simulink model "Kinematic_control"  (R2022b)
settings: Solver=FixedStepAuto  StartTime=0.0  StopTime=T_final  FixedStep=Ts  RelTol=1e-3
values from neighbouring files (symbols this model uses):
  BDD_thresh = 0.5    [Run_model.m]
  d = 0.1    [Dynamicfcn.m]    (also in Run_model.m)
  I_single = sort(randperm(n_meas,n_attack)).'    [Run_model.m]
  kx = 15    [Run_model.m]
  ky = 15    [Run_model.m]
  max_iter = 2000    [Run_model.m]
  n_meas = 6    [Run_model.m]
  P_inp = 1e-8    (= 1e-08)    [Run_model.m]
  R_meas = 1e-4    (= 0.0001)    [Run_model.m]
  T_start_attack = .2*T_final    (= 60)    [Run_model.m]
  Ts = 0.01    [Dynamicfcn.m]    (also in Run_model.m)
  u0 = zeros(n_int,1)    [Run_model.m]
  y0 = zeros(n_meas,1)    [Run_model.m]
  z_hat0 = z_initial    [Run_model.m]
  z_initial = [theta0;x0;y0]    [Run_model.m]
undefined symbols (not defined in the file or in its folder): e
libraries: simulink x3, sharedTrackingLibrary x1
settings Model: Creator=Abelb  LastModifiedBy=Abelb

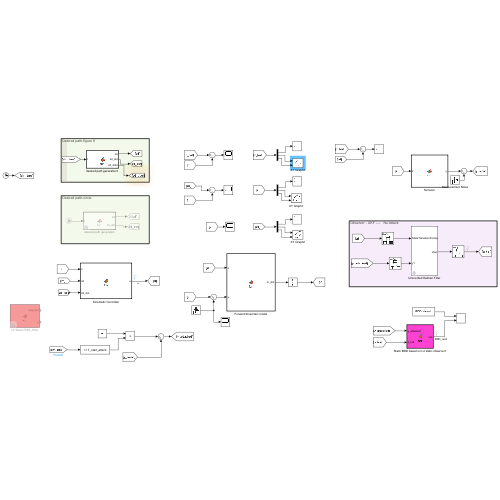
[thumbnail: Simulink's stored preview of the top-level diagram]
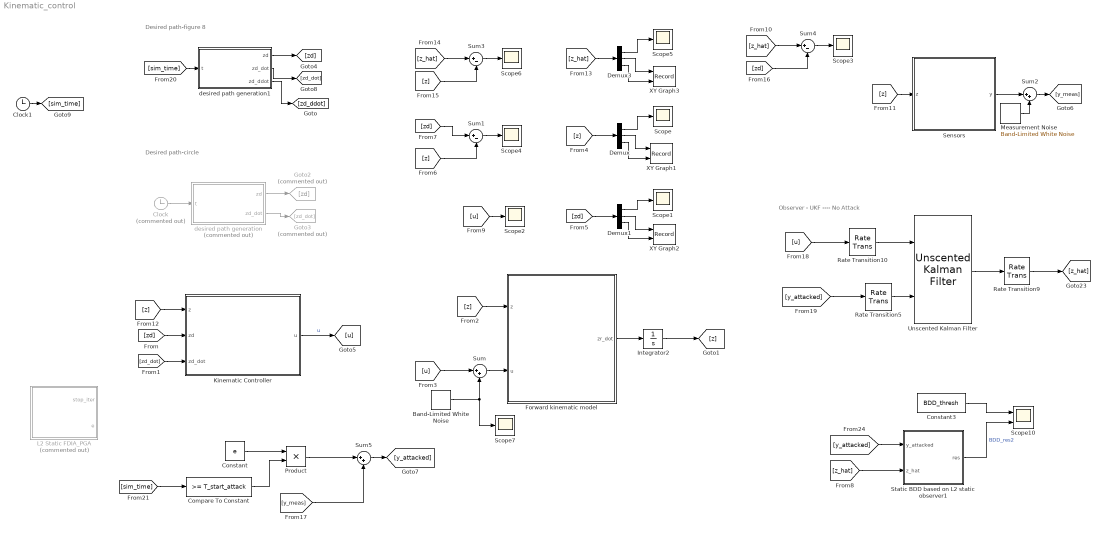
== system Kinematic_control ==
  note: Desired path-circle
  note: Desired path-figure 8
  note: Observer - UKF ---- No Attack
  Band-Limited White Noise : simulink/Sources/Band-Limited White Noise  Cov=P_inp*Ts  Ts=Ts  seed=[23341]
  Clock : Clock  Commented=on
  Clock1 : Clock
  Compare To Constant : simulink/Logic and Bit Operations/Compare To Constant  relop=>=  const=T_start_attack  OutDataTypeStr=boolean
  Constant : Constant  Value=e
  Constant3 : Constant  Value=BDD_thresh
  Demux : Demux  Outputs=3
  Demux1 : Demux  Outputs=3
  Demux3 : Demux  Outputs=3
  Forward kinematic model : MATLAB Function  TreatAsAtomicUnit=on
  Goto2 : Goto  Commented=on  GotoTag=zd
  Goto3 : Goto  Commented=on  GotoTag=zd_dot
  Integrator2 : Integrator  InitialCondition=z_initial
  Kinematic Controller : MATLAB Function  TreatAsAtomicUnit=on
  L2 Static FDIA_PGA : MATLAB Function  Commented=on  TreatAsAtomicUnit=on
  Measurement Noise : simulink/Sources/Band-Limited White Noise  Cov=R_meas*Ts  Ts=Ts  seed=[23341]
  Product : Product
  Rate Transition10 : RateTransition  InitialCondition=u0  OutPortSampleTime=Ts
  Rate Transition5 : RateTransition  InitialCondition=y0  OutPortSampleTime=Ts
  Rate Transition9 : RateTransition  InitialCondition=z_hat0  OutPortSampleTime=0
  Scope{,1..7} (8 alike) : Scope
  Scope10 : Scope  NumInputPorts=2
  Sensors : MATLAB Function  TreatAsAtomicUnit=on
  Static BDD based on L2 static observer1 : MATLAB Function  TreatAsAtomicUnit=on
  Sum : Sum  Inputs=|++
  Sum1 : Sum  Inputs=|+-
  Sum2 : Sum  Inputs=|++
  Sum3 : Sum  Inputs=|+-
  Sum4 : Sum  Inputs=|+-
  Sum5 : Sum  Inputs=|++
  Unscented Kalman Filter : sharedTrackingLibrary/Unscented Kalman Filter  StateTransitionFcn=Dynamicfcn  HasAdditiveProcessNoise=Additive  ProcessNoise=P_diag  HasTimeVaryingProcessNoise=off  HasStateTransitionFcnExtraArgument=1  InitialState=z_hat0  InitialStateCovariance=1  Alpha=1e-3  Beta=2  Kappa=0  MeasurementFcn1=measurement_model  HasMeasurementEnablePort1=off  HasAdditiveMeasurementNoise1=Additive  MeasurementNoise1=R_diag  HasTimeVaryingMeasurementNoise1=off  HasMeasurementFcnExtraArgument1=0  HasMeasurementWrapping1=off  MeasurementFcn2=myMeasurementFcn  HasMeasurementEnablePort2=off  HasAdditiveMeasurementNoise2=Additive  MeasurementNoise2=1  HasTimeVaryingMeasurementNoise2=off  HasMeasurementFcnExtraArgument2=0  HasMeasurementWrapping2=off  MeasurementFcn3=myMeasurementFcn  HasMeasurementEnablePort3=off  HasAdditiveMeasurementNoise3=Additive  MeasurementNoise3=1  HasTimeVaryingMeasurementNoise3=off  HasMeasurementFcnExtraArgument3=0  HasMeasurementWrapping3=off  MeasurementFcn4=myMeasurementFcn  HasMeasurementEnablePort4=off  HasAdditiveMeasurementNoise4=Additive  MeasurementNoise4=1  HasTimeVaryingMeasurementNoise4=off  HasMeasurementFcnExtraArgument4=0  HasMeasurementWrapping4=off  MeasurementFcn5=myMeasurementFcn  HasMeasurementEnablePort5=off  HasAdditiveMeasurementNoise5=Additive  MeasurementNoise5=1  HasTimeVaryingMeasurementNoise5=off  HasMeasurementFcnExtraArgument5=0  HasMeasurementWrapping5=off  EnableMultirate=off  StateTransitionFcnSampleTime=1  MeasurementFcn1SampleTime=1  MeasurementFcn2SampleTime=1  MeasurementFcn3SampleTime=1  MeasurementFcn4SampleTime=1  MeasurementFcn5SampleTime=1  UseCurrentEstimator=on  OutputStateCovariance=off  DataType=double  SampleTime=Ts  NumberOfMeasurements=1
      settings: LibrarySourceBlock=cstblocks/State Estimation/Unscented Kalman Filter
  XY Graph1 : Record  FileSettingsInternal="{\"entries\":[{\"content\":{\"excelSettings\":{\"content\":{},\"type\":\"Streamout.ExcelSettings\"}},\"type\":\"Streamout.FileSettingStorage\",\"uuid\":\"d8d7f9e9-d613-4e63-a397-f7a228f7e83d\"}],\"packageUris\":[\"http://schema.mathworks.com/mf0/streamout_blocks/R2020a\"],\"version\":\"1.0\"}"  Layout=[1 1]  SignalsInternal="{\"entries\":[{\"content\":{\"signals\":[{\"content\":{\"blockPath\":[\"Kinematic_control/XY Graph1\"],\"channel\":[],\"dimensions\":[1],\"domain\":\"Kinematic_control/XY Graph1\",\"lineColor\":\"#a2142f\",\"plots\":[1],\"port\":1,\"sid\":[\"\"],\"signalID\":63508,\"signalName\":\"Demux:2\"},\"type\":\"RecordBlkView.Signal\",\"uuid\":\"50b6bb6c-e09c-4804-b771-cf1436237063\"},{\"content\":{\"blockPath\":[\"Kinematic_control/XY Graph1\"],\"channel\":[],\"dimensions\":[1],\"domain\":\"Kinematic_control/XY Graph1\",\"lineColor\":\"#139fff\",\"plots\":[1],\"port\":2,\"sid\":[\"\"],\"signalID\":63512,\"signalName\":\"Demux:3\"},\"type\":\"RecordBlkView.Signal\",\"uuid\":\"32260233-ee04-4a66-bd71-a42f183323f2\"}]},\"type\":\"RecordBlkView.InputSignals\",\"uuid\":\"1d8d5054-33d6-4d2e-927d-19ce566ede83\"}],\"packageUris\":[\"http://schema.mathworks.com/mf0/streamout_blocks/R2020a\"],\"version\":\"1.0\"}"  VisualizationBindings="{\"xyplotplugin\":{\"info\":[{\"series\":[{\"bindingParametersList\":[{\"parameter\":\"X-Axis\",\"signalID\":63508,\"signalName\":\"Demux:2\"},{\"parameter\":\"Y-Axis\",\"signalID\":63512,\"signalName\":\"Demux:3\"}],\"seriesID\":26925}],\"subplotID\":1}]}}"  CompatibilityTag=XY
  XY Graph2 : Record  FileSettingsInternal="{\"entries\":[{\"content\":{\"excelSettings\":{\"content\":{},\"type\":\"Streamout.ExcelSettings\"}},\"type\":\"Streamout.FileSettingStorage\",\"uuid\":\"6c264cdc-8b0f-41a9-a26d-26fc4b96b343\"}],\"packageUris\":[\"http://schema.mathworks.com/mf0/streamout_blocks/R2020a\"],\"version\":\"1.0\"}"  Layout=[1 1]  SignalsInternal="{\"entries\":[{\"content\":{\"signals\":[{\"content\":{\"blockPath\":[\"Kinematic_control/XY Graph2\"],\"channel\":[],\"dimensions\":[1],\"domain\":\"Kinematic_control/XY Graph2\",\"lineColor\":\"#a2142f\",\"plots\":[1],\"port\":1,\"sid\":[\"\"],\"signalID\":63516,\"signalName\":\"Demux1:2\"},\"type\":\"RecordBlkView.Signal\",\"uuid\":\"dce2a075-dfc9-47ac-9e8c-4f7c2265c200\"},{\"content\":{\"blockPath\":[\"Kinematic_control/XY Graph2\"],\"channel\":[],\"dimensions\":[1],\"domain\":\"Kinematic_control/XY Graph2\",\"lineColor\":\"#139fff\",\"plots\":[1],\"port\":2,\"sid\":[\"\"],\"signalID\":63520,\"signalName\":\"Demux1:3\"},\"type\":\"RecordBlkView.Signal\",\"uuid\":\"2ac57c94-c318-4a92-bba8-431307e380f6\"}]},\"type\":\"RecordBlkView.InputSignals\",\"uuid\":\"2930b6aa-ee4b-4578-8e5b-7c11aa3c476f\"}],\"packageUris\":[\"http://schema.mathworks.com/mf0/streamout_blocks/R2020a\"],\"version\":\"1.0\"}"  VisualizationBindings="{\"xyplotplugin\":{\"info\":[{\"series\":[{\"bindingParametersList\":[{\"parameter\":\"X-Axis\",\"signalID\":63516,\"signalName\":\"Demux1:2\"},{\"parameter\":\"Y-Axis\",\"signalID\":63520,\"signalName\":\"Demux1:3\"}],\"seriesID\":33144}],\"subplotID\":1}]}}"  CompatibilityTag=XY
  XY Graph3 : Record  FileSettingsInternal="{\"entries\":[{\"content\":{\"excelSettings\":{\"content\":{},\"type\":\"Streamout.ExcelSettings\"}},\"type\":\"Streamout.FileSettingStorage\",\"uuid\":\"dbd449c8-5eee-492b-8755-63c5154b06c6\"}],\"packageUris\":[\"http://schema.mathworks.com/mf0/streamout_blocks/R2020a\"],\"version\":\"1.0\"}"  Layout=[1 1]  SignalsInternal="{\"entries\":[{\"content\":{\"signals\":[{\"content\":{\"blockPath\":[\"Kinematic_control/XY Graph3\"],\"channel\":[],\"dimensions\":[1],\"domain\":\"Kinematic_control/XY Graph3\",\"lineColor\":\"#a2142f\",\"plots\":[1],\"port\":1,\"sid\":[\"\"],\"signalID\":63524,\"signalName\":\"Demux3:2\"},\"type\":\"RecordBlkView.Signal\",\"uuid\":\"623d89f1-b4d6-49ba-b202-f47227c3b43a\"},{\"content\":{\"blockPath\":[\"Kinematic_control/XY Graph3\"],\"channel\":[],\"dimensions\":[1],\"domain\":\"Kinematic_control/XY Graph3\",\"lineColor\":\"#139fff\",\"plots\":[1],\"port\":2,\"sid\":[\"\"],\"signalID\":63528,\"signalName\":\"Demux3:3\"},\"type\":\"RecordBlkView.Signal\",\"uuid\":\"09bcd7e8-baa0-4f7a-91d9-299976939700\"}]},\"type\":\"RecordBlkView.InputSignals\",\"uuid\":\"2682f2ed-8ed1-4b26-a615-09d838c32bc9\"}],\"packageUris\":[\"http://schema.mathworks.com/mf0/streamout_blocks/R2020a\"],\"version\":\"1.0\"}"  VisualizationBindings="{\"xyplotplugin\":{\"info\":[{\"series\":[{\"bindingParametersList\":[{\"parameter\":\"X-Axis\",\"signalID\":63524,\"signalName\":\"Demux3:2\"},{\"parameter\":\"Y-Axis\",\"signalID\":63528,\"signalName\":\"Demux3:3\"}],\"seriesID\":8579}],\"subplotID\":1}]}}"  CompatibilityTag=XY
  desired path generation : MATLAB Function  Commented=on  TreatAsAtomicUnit=on
  desired path generation1 : MATLAB Function  TreatAsAtomicUnit=on
  wires:
  Forward kinematic model/1(zr_dot) -> Integrator2/1
  desired path generation1/3(zd_ddot) -> [zd_ddot]
  desired path generation1/2(zd_dot) -> [zd_dot]
  desired path generation1/1(zd) -> [zd]
  desired path generation/2(zd_dot) -> Goto3/1
  desired path generation/1(zd) -> Goto2/1
  Clock/1 -> desired path generation/1(t)
  [zd] -> Kinematic Controller/2(zd)
  [zd_dot] -> Kinematic Controller/3(zd_dot)
  Integrator2/1 -> [z]
  [z] -> Forward kinematic model/1(z)
  [z] -> Demux/1
  Demux/1 -> Scope/1
  Demux/2 -> XY Graph1/1
  Demux/3 -> XY Graph1/2
  Demux1/2 -> XY Graph2/1
  Demux1/3 -> XY Graph2/2
  [zd] -> Demux1/1
  Demux1/1 -> Scope1/1
  Kinematic Controller/1(u) -> [u]  "u"
  [zd] -> Sum1/1
  [z] -> Sum1/2
  Sum1/1 -> Scope4/1
  Unscented Kalman Filter/1 -> Rate Transition9/1
  Rate Transition9/1 -> [z_hat]
  Rate Transition10/1 -> Unscented Kalman Filter/1
  Rate Transition5/1 -> Unscented Kalman Filter/2
  [u] -> Rate Transition10/1
  [u] -> Scope2/1
  [z] -> Sensors/1(z)
  Measurement Noise/1 -> Sum2/2
  Demux3/2 -> XY Graph3/1
  Demux3/1 -> Scope5/1
  Demux3/3 -> XY Graph3/2
  [z_hat] -> Demux3/1
  [z] -> Sum3/2
  [z_hat] -> Sum3/1
  Sum3/1 -> Scope6/1
  [y_attacked] -> Rate Transition5/1
  Sensors/1(y) -> Sum2/1
  Sum2/1 -> [y_meas]
  Sum4/1 -> Scope3/1
  [zd] -> Sum4/2
  [z_hat] -> Sum4/1
  [z] -> Kinematic Controller/1(z)
  Sum/1 -> Forward kinematic model/2(u)
  [u] -> Sum/1
  Band-Limited White Noise/1 -> Scope7/1, Sum/2
  [y_meas] -> Sum5/2
  Sum5/1 -> [y_attacked]
  Product/1 -> Sum5/1
  Clock1/1 -> [sim_time]
  [sim_time] -> desired path generation1/1(t)
  [sim_time] -> Compare To Constant/1
  Compare To Constant/1 -> Product/2
  Constant/1 -> Product/1
  [y_attacked] -> Static BDD based on L2 static observer1/1(y_attacked)
  Constant3/1 -> Scope10/1
  [z_hat] -> Static BDD based on L2 static observer1/2(z_hat)
  Static BDD based on L2 static observer1/1(res) -> Scope10/2  "BDD_res2"

== matlab function Kinematic_control/desired path generation1 ==
  data: t input; zd output; zd_dot output; zd_ddot output
function [zd,zd_dot,zd_ddot] = fcn(t)

t = t/10;

a=1;
x = a*cos(t)/(1+sin(t)^2);
y = a*sin(t)*cos(t)/(1+sin(t)^2);
% unit circle (radius = 1; origin: (0,0))
zd = [atan(y./x);              % theta
      a*cos(t)/(1+sin(t)^2);         % x
      a*sin(t)*cos(t)/(1+sin(t)^2)];        % y

zd_dot = [ 0;
          -a*sin(t)*(cos(t)^2+2)/(1+sin(t)^2)^2;
          (a*cos(t)^2-2*a*sin(t)^2)/(1+sin(t)^2)^2];

z1 = (a*sin(t)^2*cos(t)^3-11*a*cos(t)^3+8*a*cos(t))/(1+sin(t)^2)^3;
z2 = -2*a*sin(t)*cos(t)*(3+2*cos(t)^2-sin(t)^2)/(1+sin(t)^2)^3;
zd_ddot = [z1;
           z2];

== matlab function Kinematic_control/Kinematic Controller ==
  data: z input; u output; zd input; zd_dot input; d parameter; kx parameter; ky parameter
function u = fcn(z,zd,zd_dot,d, kx, ky)

%% unpacking inputs
theta = z(1);
x = z(2);
y = z(3);
xd = zd(2);
yd = zd(3);
xd_dot = zd_dot(2);
yd_dot = zd_dot(3);



%% controller
K1 = [cos(theta) sin(theta);
     -sin(theta)/d cos(theta)/d];
K2 = [xd_dot + kx*(xd-x) ;
      yd_dot + ky*(yd-y)];
u = K1*K2;



%% rate constraint (physics)
v = u(1);
omega = u(2);

%% packing output
u = [v;
     omega];

== matlab function Kinematic_control/Sensors ==
  data: z input; y output; n_meas parameter
function y = fcn(z,n_meas)

coder.extrinsic('measurement_model');

y = zeros(n_meas,1);
y(:) = measurement_model(z);

== matlab function Kinematic_control/Forward kinematic model ==
  data: z input; u input; zr_dot output; d parameter
function zr_dot = fcn(z,u,d)

%% unpacking the state vectors
theta=z(1);

%% unpacking the intput
v=u(1);
omega=u(2);

%% ODE
theta_dot=omega;
x_dot=v*cos(theta)-d*omega*sin(theta);
y_dot=v*sin(theta)+d*omega*cos(theta);
% phir_dot = (v+omega)/r;
% phil_dot = (v-omega)/r;


%% packing the output
zr_dot=[theta_dot;x_dot;y_dot];

== matlab function Kinematic_control/L2 Static FDIA_PGA ==
  data: stop_iter output; I_single parameter; e output; BDD_thresh parameter; max_iter parameter; n_meas parameter
function [stop_iter,e]  = fcn(I_single,BDD_thresh,max_iter, n_meas)

coder.extrinsic('L2_FDIA2');
%% Measurement Channel Attack
%  Assumptions:
%  1. The attacker knows the actual measurement
%  2. The attacker can only corrupt upto n_attack measurements
%  3. The attacker knows the BDD theshold

attack_idx = I_single;
% e = L2_FDIA(C_obsv_d,attack_idx,0.9*BDD_thresh);

L=0.235/2;  %1/2 distance between two wheels,(m)
r=0.05;     %radius of wheels,(m)

C = @(x,y,theta) [-x*sin(theta) cos(theta) 0;
                   y*cos(theta) 0 sin(theta);
                   0 1 0;
                   0 0 1;
                   0 1/(4*r) L/(4*r);
                   0 1/(4*r) -L/(4*r)];
Cd = C(1.5, 1, 0);

e = zeros(n_meas,1);
stop_iter = 0;
[stop_iter(:),e(:)] = L2_FDIA2(Cd,attack_idx,BDD_thresh,max_iter);

== matlab function Kinematic_control/desired path generation ==
  data: t input; zd output; zd_dot output
function [zd,zd_dot] = fcn(t)

 t = t/10;


% unit circle (radius = 1; origin: (0,0))
zd = [t;
      sin(t);         % x
      -1*cos(t)];        % y

zd_dot = [1;
          1*cos(t) ;
          1*sin(t) ];

== matlab function Kinematic_control/Static BDD based on L2 static observer1 ==
  data: y_attacked input; z_hat input; res output; n_meas parameter
function res = fcn(y_attacked,z_hat,n_meas)

coder.extrinsic('measurement_model');

y = zeros(n_meas,1);
y(:) = measurement_model(z_hat);

res = norm(y_attacked-y,2);
